simulink model "motor"  (R2015a)
settings: Solver=ode45  StartTime=0.0  StopTime=20  RelTol=1e-3
values from neighbouring files (symbols this model uses):
  b = 0.001    [sim_DC.m]
  i = 210/15    (= 14)    [sim_DC.m]
  J = J_mass/(i^2)    (= 0.00510204081633)    [sim_DC.m]
  K_e = 0.147    [sim_DC.m]
  K_t = 0.147    [sim_DC.m]
  L = 0.82e-3    (= 0.00082)    [sim_DC.m]
  R = 1.03    [sim_DC.m]
  r = 0.1    [sim_DC.m]
  V = 10    [sim_DC.m]
settings Model: CovSFcnEnable=off  Creator=joojala2  LastModifiedBy=tlantela

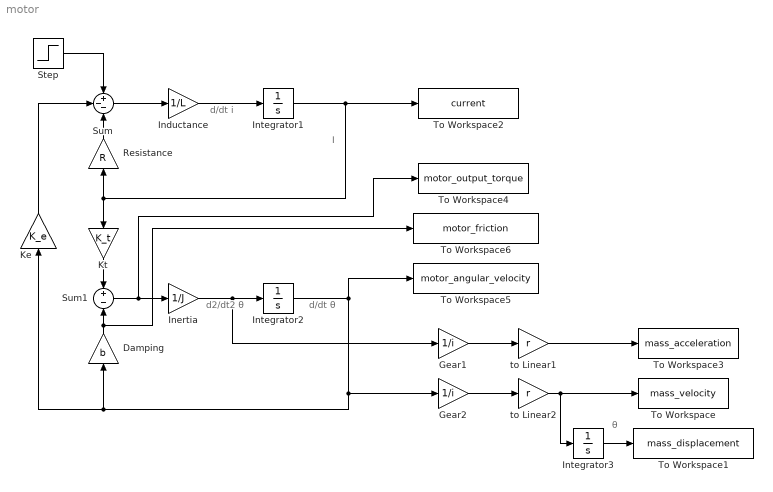
== system motor ==
  note: d/dt i
  note: I
  note: d2/dt2 θ
  note: d/dt θ
  note: θ
  Damping : Gain  Gain=b
  Gear1 : Gain  Gain=1/i
  Gear2 : Gain  Gain=1/i
  Inductance : Gain  Gain=1/L
  Inertia : Gain  Gain=1/J
  Integrator1 : Integrator
  Integrator2 : Integrator
  Integrator3 : Integrator
  Ke : Gain  Gain=K_e
  Kt : Gain  Gain=K_t
  Resistance : Gain  Gain=R
  Step : Step  Time=0  After=V  SampleTime=1
  Sum : Sum  Inputs=+--
  Sum1 : Sum  Inputs=+|-
  To Workspace : ToWorkspace  VariableName=mass_velocity  SaveFormat=Timeseries  SampleTime=-1
  To Workspace1 : ToWorkspace  VariableName=mass_displacement  SaveFormat=Timeseries  SampleTime=-1
  To Workspace2 : ToWorkspace  VariableName=current  SaveFormat=Timeseries  SampleTime=-1
  To Workspace3 : ToWorkspace  VariableName=mass_acceleration  SaveFormat=Timeseries  SampleTime=-1
  To Workspace4 : ToWorkspace  VariableName=motor_output_torque  SaveFormat=Timeseries  SampleTime=-1
  To Workspace5 : ToWorkspace  VariableName=motor_angular_velocity  SaveFormat=Timeseries  SampleTime=-1
  To Workspace6 : ToWorkspace  VariableName=motor_friction  SaveFormat=Timeseries  SampleTime=-1
  to Linear1 : Gain  Gain=r
  to Linear2 : Gain  Gain=r
  wires:
  Integrator2/1 -> Gear2/1, Damping/1, Ke/1, To Workspace5/1
  Damping/1 -> To Workspace6/1, Sum1/2
  Sum1/1 -> To Workspace4/1, Inertia/1
  Kt/1 -> Sum1/1
  Ke/1 -> Sum/2
  Resistance/1 -> Sum/3
  Step/1 -> Sum/1
  Inertia/1 -> Gear1/1, Integrator2/1
  Inductance/1 -> Integrator1/1
  Sum/1 -> Inductance/1
  Integrator1/1 -> To Workspace2/1, Kt/1, Resistance/1
  Gear1/1 -> to Linear1/1
  to Linear1/1 -> To Workspace3/1
  Gear2/1 -> to Linear2/1
  to Linear2/1 -> Integrator3/1, To Workspace/1
  Integrator3/1 -> To Workspace1/1
